simulink model "HarmonicSeriesRecreation2"  (R2021a)
settings: Solver=FixedStepAuto  StartTime=0.0  StopTime=1  FixedStep=1/44100  RelTol=1e-3
libraries: dspsnks4 x1, dspvision x1
settings Model: Creator=ZZDDD  LastModifiedBy=ZZDDD

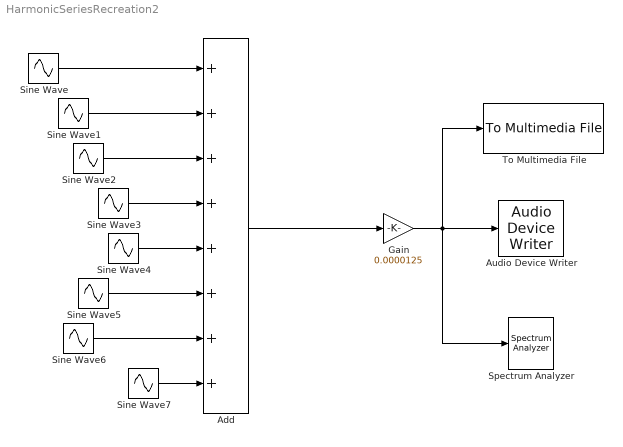
== system HarmonicSeriesRecreation2 ==
  Add : Sum  Inputs=++++++++
  Audio Device Writer : dspsnks4/Audio Device Writer  Driver=DirectSound  Device=Default  InheritSampleRate=on  SampleRate=44100  BitDepth=16-bit integer  BufferSize=4096  NumBuffers=10  DefaultOutputChannelMapping=on  OutputChannelMapping=1:2  OutputNumUnderrunSamples=off  DriverIdx=1  DeviceWarnFlag=''
  Gain : Gain  Gain=0.0000125  OutDataTypeStr=Inherit: Same as input
  Sine Wave : Sin  Amplitude=5357  Frequency=440 * 2 * pi  SampleTime=1/44100
  Sine Wave1 : Sin  Amplitude=1048.8  Frequency=440 * 2 * pi * 2  SampleTime=1/44100
  Sine Wave2 : Sin  Amplitude=494.3  Frequency=440 * 2 * pi * 3  SampleTime=1/44100
  Sine Wave3 : Sin  Amplitude=89  Frequency=440 * 2 * pi * 4  SampleTime=1/44100
  Sine Wave4 : Sin  Amplitude=61.2  Frequency=440 * 2 * pi * 5  SampleTime=1/44100
  Sine Wave5 : Sin  Amplitude=108.97  Frequency=440 * 2 * pi * 6  SampleTime=1/44100
  Sine Wave6 : Sin  Amplitude=3.27  Frequency=440 * 2 * pi * 7  SampleTime=1/44100
  Sine Wave7 : Sin  Amplitude=26.7  Frequency=440 * 2 * pi * 8  SampleTime=1/44100
  Spectrum Analyzer : SpectrumAnalyzer
  To Multimedia File : dspvision/To Multimedia File  outputFilename=C:\Users\ZZDDD\OneDrive\基础物理实验\Simulink Analysis & Recreation Harmonic Series\output.wav  streamSelection=Audio only  videoCompressor=None (uncompressed)  audioCompressor=None (uncompressed)  imagePorts=Separate color signals  fileType=WAV  audioDatatype=16-bit integer  fourcc=RGB  videoQuality=75  mj2000CompFactor=10
  wires:
  Sine Wave/1 -> Add/1
  Sine Wave7/1 -> Add/8
  Sine Wave6/1 -> Add/7
  Sine Wave5/1 -> Add/6
  Sine Wave4/1 -> Add/5
  Sine Wave3/1 -> Add/4
  Sine Wave2/1 -> Add/3
  Sine Wave1/1 -> Add/2
  Add/1 -> Gain/1
  Gain/1 -> To Multimedia File/1, Spectrum Analyzer/1, Audio Device Writer/1
